simulink model "simulator_prototype"  (R2021b)
settings: Solver=VariableStepAuto  StartTime=0.0  StopTime=200  FixedStep=0.01  RelTol=1e-3
StopFcn:
  | run('simulate_robot_plot3.m')
(part 3 of 12)

== matlab function simulator_prototype/Kinematic Model/foward_kinematics ==
  data: q1 input; fk0_6 output; q2 input; q3 input; q4 input; q5 input; q6 input
function fk0_6 = foward_kinematics(q1,q2,q3,q4,q5,q6)
%#codegen

%    This function was generated by the Symbolic Math Toolbox version 9.0.
%    10-Oct-2021 02:08:10

t2 = cos(q1);
t3 = cos(q2);
t4 = cos(q4);
t5 = cos(q5);
t6 = cos(q6);
t7 = sin(q1);
t8 = sin(q2);
t9 = sin(q4);
t10 = sin(q5);
t11 = sin(q6);
t12 = q1+q2;
t23 = 9.007199254740992e+15;
t13 = cos(t12);
t14 = sin(t12);
t20 = t2.*1.051339e-1;
t21 = t7.*1.051339e-1;
t22 = t7.*3.235525e-2;
t24 = t2.*3.235525e-2;
t26 = t2.*t3.*3.641522e-2;
t27 = t2.*t8.*3.641522e-2;
t28 = t3.*t7.*3.641522e-2;
t29 = t7.*t8.*3.641522e-2;
t30 = t7.*t8.*2.462267e-2;
t32 = t2.*t3.*2.462267e-2;
t33 = t2.*t8.*2.462267e-2;
t34 = t3.*t7.*2.462267e-2;
t38 = (q3.*t23)./9.007199254740992e+15;
t41 = q3.*t23.*1.110223024625157e-16i;
t15 = t14.*7.742227997977903e+15;
t16 = t13.*4.602992943936994e+15;
t17 = t14.*4.602992943936994e+15;
t18 = t13.*7.742227997977903e+15;
t25 = -t22;
t31 = -t26;
t35 = -t30;
t39 = cos(t38);
t40 = sin(t38);
t42 = exp(t41);
t43 = -t41;
t19 = -t17;
t36 = t15+t16;
t44 = 1.0./t42;
t45 = t4.*t39;
t46 = t9.*t39;
t47 = t40.*1i;
t48 = t42-1.0;
t53 = t39.*7.38843356682345e-1;
t54 = t39.*2.61156643317655e-1;
t56 = t23.*t40.*9.543032792050485e-17;
t57 = t4.*t23.*t40.*5.673626844500105e-17;
t58 = t9.*t23.*t40.*5.673626844500105e-17;
t62 = t5.*t23.*t40.*(-9.543032792050485e-17);
t65 = t4.*t23.*t40.*(t17-t18).*(-1.232595164407831e-32);
t67 = t9.*t23.*t40.*(t17-t18).*(-1.232595164407831e-32);
t68 = (t4.*t23.*t40.*(t17-t18))./8.112963841460668e+31;
t69 = (t9.*t23.*t40.*(t17-t18))./8.112963841460668e+31;
t70 = t23.*t40.*5.540299264978165e-18;
t37 = t18+t19;
t49 = -t47;
t50 = t48.^2;
t52 = t39+t47-1.0;
t59 = t5.*t56;
t60 = t10.*t56;
t61 = -t58;
t63 = (t4.*t23.*t36.*t40)./8.112963841460668e+31;
t64 = (t9.*t23.*t36.*t40)./8.112963841460668e+31;
t71 = t53+2.61156643317655e-1;
t72 = t54+7.38843356682345e-1;
t77 = t46+t57;
t51 = t39+t49;
t55 = t52.^2;
t66 = -t64;
t73 = t13.*t71;
t74 = t13.*t72;
t75 = t14.*t71;
t76 = t14.*t72;
t78 = t45+t61;
t79 = t5.*t78;
t80 = t10.*t78;
t81 = t13.*t51.*t55.*2.196325630278387e-1;
t82 = t14.*t51.*t55.*2.196325630278387e-1;
t83 = -t81;
t84 = -t82;
t85 = t60+t79;
t86 = t62+t80;
t87 = t74+t82;
t88 = t75+t81;
t89 = t73+t84;
t90 = t76+t83;
t91 = t4.*t87;
t92 = t5.*t88;
t93 = t9.*t87;
t94 = t10.*t88;
t95 = t4.*t90;
t96 = t5.*t89;
t97 = t9.*t90;
t98 = t10.*t89;
t100 = t63+t93;
t101 = t66+t91;
t99 = -t95;
t102 = t67+t95;
t103 = t68+t97;
t104 = t5.*t100;
t105 = t10.*t100;
t106 = t69+t99;
t107 = -t104;
t108 = t5.*t103;
t109 = t10.*t103;
t111 = t92+t105;
t110 = -t109;
t112 = t94+t107;
t113 = t98+t108;
t114 = t96+t110;
et1 = t21+t24-t2.*t3.*5.561103841189621e-2;
et2 = t2.*t8.*3.603517512464e-2;
et3 = t3.*t7.*3.603517512464e-2;
et4 = t7.*t8.*5.561103841189621e-2;
et5 = t2.*t3.*t39.*6.463878411896211e-3;
et6 = t2.*t8.*t39.*1.087223487536e-2;
et7 = t3.*t7.*t39.*1.087223487536e-2;
et8 = t7.*t8.*t39.*(-6.463878411896211e-3);
et9 = t20+t25+t2.*t3.*3.603517512464e-2;
et10 = t2.*t8.*5.561103841189621e-2;
et11 = t3.*t7.*5.561103841189621e-2;
et12 = t7.*t8.*(-3.603517512464e-2);
et13 = t2.*t3.*t39.*1.087223487536e-2;
et14 = t2.*t8.*t39.*(-6.463878411896211e-3);
et15 = t3.*t7.*t39.*(-6.463878411896211e-3);
et16 = t7.*t8.*t39.*(-1.087223487536e-2);
et17 = t21+t24-t2.*t3.*7.464911842399381e-2;
et18 = t2.*t8.*4.735389991350965e-2;
et19 = t3.*t7.*4.735389991350965e-2;
et20 = t7.*t8.*7.464911842399381e-2;
et21 = t2.*t3.*t39.*2.550195842399381e-2;
et22 = t2.*t8.*t39.*4.289426008649035e-2;
et23 = t3.*t7.*t39.*4.289426008649035e-2;
et24 = t7.*t8.*t39.*(-2.550195842399381e-2);
et25 = t20+t25+t2.*t3.*4.735389991350965e-2;
et26 = t2.*t8.*7.464911842399381e-2;
et27 = t3.*t7.*7.464911842399381e-2;
et28 = t7.*t8.*(-4.735389991350965e-2);
et29 = t2.*t3.*t39.*4.289426008649035e-2;
et30 = t2.*t8.*t39.*(-2.550195842399381e-2);
et31 = t3.*t7.*t39.*(-2.550195842399381e-2);
et32 = t7.*t8.*t39.*(-4.289426008649035e-2);
et33 = t21+t24+t29+t31+t33+t34-t74.*1.273194e-2+t75.*6.562549e-2+t92.*(3.0./5.0e+2)+t105.*(3.0./5.0e+2)+t13.*t44.*t50.*1.44134945686578e-2;
et34 = t14.*t44.*t50.*(-2.79634861451666e-3);
et35 = t20+t25+t27+t28+t32+t35+t73.*6.562549e-2+t76.*1.273194e-2+t96.*(3.0./5.0e+2)-t109.*(3.0./5.0e+2)-t13.*t44.*t50.*2.79634861451666e-3;
et36 = t14.*t44.*t50.*(-1.44134945686578e-2);
mt1 = [t2,t13,t87,t101,t101,-t11.*t111-t6.*(t64-t91),0.0,0.0,t23.*t40.*5.673626844500105e-17,t77,t77,t6.*t77+t11.*t86,-t7,-t14,-t76+t81,t106,t106,-t6.*t102-t11.*t114,0.0,0.0,0.0,0.0,0.0,0.0,0.0,0.0,t23.*t36.*t40.*(-1.232595164407831e-32),-t100,t112,t112,1.0,1.0,t39,t78,t85,t85,0.0,0.0];
mt2 = [(t23.*t40.*(t17-t18))./8.112963841460668e+31,t103,t113,t113,0.0,0.0,0.0,0.0,0.0,0.0,t7,t14,t88,t88,t111,t6.*t111-t11.*(t64-t91),0.0,0.0,t56,t56,t59-t80,t11.*t77-t6.*t86,t2,t13,t89,t89,t114,-t11.*t102+t6.*t114,0.0,0.0,0.0,0.0,0.0,0.0,0.0,t21+t24,t21+t24+t29+t31+t33+t34,et1+et2+et3+et4+et5+et6+et7+et8,et17+et18+et19+et20+et21+et22+et23+et24,et33+et34,0.0,0.0,0.0];
mt3 = [t23.*t40.*1.404277280157545e-18,t70,t70-t80.*(3.0./5.0e+2)+t5.*t23.*t40.*5.725819675230291e-19,0.0,t20+t25,t20+t25+t27+t28+t32+t35,et9+et10+et11+et12+et13+et14+et15+et16,et25+et26+et27+et28+et29+et30+et31+et32,et35+et36,1.0,1.0,1.0,1.0,1.0,1.0];
fk0_6 = reshape([mt1,mt2,mt3],6,16);

== matlab function simulator_prototype/Kinematic Model/MATLAB Function ==
  data: fk_0_6 input; coord output
function coord = fcn(fk_0_6)
    coord = zeros(size(fk_0_6, 1),3);
    for i = 1:size(fk_0_6, 1)
        h_i = reshape(fk_0_6(i,:),4,4);
        coord(i,:) = real(h_i(1:3,4)');
    end

end

== matlab function simulator_prototype/Dynamic Model/Gravity_vector ==
  data: q1 input; tau_g output; q2 input; q3 input; q4 input; q5 input; q6 input
function tau_g = Gravity_vector(q1,q2,q3,q4,q5,q6)
%#codegen

%    This function was generated by the Symbolic Math Toolbox version 9.0.
%    08-Oct-2021 20:02:44

t2 = conj(q1);
t3 = conj(q2);
t4 = conj(q3);
t5 = conj(q4);
t6 = conj(q5);
t7 = conj(q6);
t23 = atan(5.945307920587191e-1);
t24 = 9.007199254740992e+15;
t8 = cos(t2);
t9 = cos(t3);
t10 = cos(t5);
t11 = cos(t6);
t12 = cos(t7);
t13 = sin(t2);
t14 = sin(t3);
t15 = sin(t5);
t16 = sin(t6);
t17 = sin(t7);
t18 = t2+t3;
t28 = (t4.*t24)./9.007199254740992e+15;
t31 = t4.*t24.*1.110223024625157e-16i;
t19 = cos(t18);
t20 = sin(t18);
t25 = t18+t23;
t29 = cos(t28);
t30 = sin(t28);
t32 = -t31;
t33 = exp(t31);
t21 = t19.*4.602992943936994e+15;
t22 = t20.*7.742227997977903e+15;
t26 = sin(t25);
t34 = -t29;
t35 = exp(t32);
t36 = t30.*1i;
t37 = t10.*t29;
t38 = t15.*t29;
t45 = t29.*7.38843356682345e-1;
t46 = t29.*2.61156643317655e-1;
t49 = t10.*t24.*t30.*5.673626844500105e-17;
t50 = t15.*t24.*t30.*5.673626844500105e-17;
t51 = t11.*t24.*t30.*9.543032792050485e-17;
t65 = t8.*t9.*t29.*4.598452461113469e-3;
t66 = t13.*t14.*t29.*4.598452461113469e-3;
t68 = t8.*t14.*t29.*7.73459091191916e-3;
t69 = t9.*t13.*t29.*7.73459091191916e-3;
t27 = t21+t22;
t39 = t35-1.0;
t41 = t15.*t26.*t30;
t42 = t10.*t26.*t30;
t44 = t29+t36;
t47 = t34+t36+1.0;
t52 = -t50;
t53 = -t51;
t61 = t45+2.61156643317655e-1;
t62 = t46+7.38843356682345e-1;
t67 = -t65;
t70 = -t68;
t71 = -t69;
t72 = t38+t49;
t40 = t39.^2;
t43 = -t41;
t48 = t47.^2;
t54 = t42.*1.834077274308e-6;
t56 = t41.*1.663769266031448e-3;
t57 = (t10.*t24.*t27.*t30)./8.112963841460668e+31;
t58 = (t15.*t24.*t27.*t30)./8.112963841460668e+31;
t63 = t19.*t62;
t64 = t20.*t61;
t73 = t37+t52;
t55 = -t54;
t59 = -t56;
t60 = -t58;
t74 = t16.*t73;
t75 = t20.*t33.*t40.*1.993592526573721e-4;
t76 = t63.*9.0769442339979e-4;
t77 = t64.*1.123016940370151e-2;
t78 = t19.*t33.*t40.*1.027576994682181e-3;
t81 = t20.*t44.*t48.*2.196325630278387e-1;
t82 = t19.*t44.*t48.*2.196325630278387e-1;
t84 = t19.*t44.*t48.*1.438933894689597e-3;
t79 = -t77;
t80 = -t78;
t83 = t53+t74;
t85 = -t84;
t86 = t63+t81;
t87 = t64+t82;
t88 = t10.*t86;
t89 = t11.*t87;
t90 = t15.*t86;
t91 = t16.*t87.*1.33075164870018e-3;
t92 = -t91;
t93 = t90.*1.834077274308e-6;
t95 = t88.*1.663769266031448e-3;
t96 = t89.*1.03455776890854e-3;
t98 = t42+t90;
t99 = t43+t88;
t102 = t12.*(t41-t88).*(-7.12549896598485e-4);
t103 = t57+t90;
t104 = t60+t88;
t105 = t17.*(t41-t88).*(-1.31098441441266e-3);
t106 = t17.*(t41-t88).*1.31098441441266e-3;
t94 = -t93;
t97 = -t96;
t100 = t16.*t98;
t101 = t11.*t98.*1.33075164870018e-3;
t108 = t16.*t103;
t107 = t100.*1.03455776890854e-3;
t110 = t89+t100;
t115 = t89+t108;
t109 = -t107;
t111 = t17.*t110.*7.12549896598485e-4;
t113 = t12.*t110.*1.31098441441266e-3;
t112 = -t111;
t114 = -t113;
et1 = t8.*(-1.504629097027635e-2)-t13.*3.4643831698033e-2;
et2 = t19.*4.486342129859745e-3-t20.*3.161090981652867e-3+t55+t59+t66+t67+t70+t71+t75+t76+t79+t80+t85+t92+t94+t95+t97+t101+t102+t106+t109+t112+t114;
et3 = t8.*t9.*2.789883597074818e-2;
et4 = t8.*t14.*(-1.805586507105727e-2);
et5 = t9.*t13.*(-1.805586507105727e-2);
et6 = t13.*t14.*(-2.789883597074818e-2);
et7 = t19.*(-1.035229938014282e-2)+t20.*7.294263179826428e-3+t55+t59+t66+t67+t70+t71+t75+t76+t79+t80+t85+t92+t94+t95+t97+t101+t102+t106+t109+t112+t114;
et8 = t8.*t9.*2.716427583908298e-2;
et9 = t8.*t14.*(-1.753829165813497e-2);
et10 = t9.*t13.*(-1.753829165813497e-2);
et11 = t13.*t14.*(-2.716427583908298e-2);
et12 = t37.*-6.451751339289925e+65-t38.*5.852657213932193e+68;
et13 = t11.*t37.*4.681197925536181e+68-t12.*t38.*2.506543652270432e+68;
et14 = t16.*t37.*-3.639273854285582e+68+t24.*t30.*6.584058839489303e+53;
et15 = t17.*t38.*4.611662534593243e+68-t10.*t24.*t30.*3.320579308062288e+52+t11.*t24.*t30.*3.472970973069927e+52;
et16 = t12.*t16.*t37.*-4.611662534593243e+68+t15.*t24.*t30.*3.660482959263482e+49;
et17 = t16.*t17.*t37.*-2.506543652270432e+68+t16.*t24.*t30.*4.467282530947048e+52-t10.*t12.*t24.*t30.*1.422119335243286e+52;
et18 = t11.*t12.*t24.*t30.*4.400924679349397e+52-t11.*t15.*t24.*t30.*2.655937021474028e+52+t10.*t17.*t24.*t30.*2.616485235404362e+52;
et19 = t11.*t17.*t24.*t30.*2.392002826832272e+52+t15.*t16.*t24.*t30.*2.064788183416204e+52+t12.*t15.*t16.*t24.*t30.*2.616485235404362e+52;
et20 = t15.*t16.*t17.*t24.*t30.*1.422119335243286e+52;
et21 = t8.*t9.*t10.*5.058701277356498e-7;
et22 = t8.*t9.*t15.*4.539519387384721e-4;
et23 = t8.*t10.*t14.*8.508728807534787e-7;
et24 = t9.*t10.*t13.*8.508728807534787e-7;
et25 = t8.*t14.*t15.*7.635465560438749e-4;
et26 = t9.*t13.*t15.*7.635465560438749e-4;
et27 = t10.*t13.*t14.*(-5.058701277356498e-7);
et28 = t13.*t14.*t15.*(-4.539519387384721e-4);
et29 = t8.*t9.*t10.*t11.*5.84552790715085e-4;
et30 = t8.*t9.*t10.*t16.*(-4.544451487714901e-4);
et31 = t8.*t10.*t11.*t14.*9.832170150362058e-4;
et32 = t9.*t10.*t11.*t13.*9.832170150362058e-4;
et33 = t8.*t9.*t12.*t15.*(-3.129983201502934e-4);
et34 = t8.*t10.*t14.*t16.*(-7.643761346621835e-4);
et35 = t9.*t10.*t13.*t16.*(-7.643761346621835e-4);
et36 = t10.*t11.*t13.*t14.*(-5.84552790715085e-4);
et37 = t8.*t9.*t15.*t17.*5.758697340540054e-4;
et38 = t8.*t12.*t14.*t15.*(-5.264627574064825e-4);
et39 = t9.*t12.*t13.*t15.*(-5.264627574064825e-4);
et40 = t10.*t13.*t14.*t16.*4.544451487714901e-4;
et41 = t8.*t14.*t15.*t17.*9.686121253028882e-4;
et42 = t9.*t13.*t15.*t17.*9.686121253028882e-4;
et43 = t12.*t13.*t14.*t15.*3.129983201502934e-4;
et44 = t13.*t14.*t15.*t17.*(-5.758697340540054e-4);
et45 = t8.*t9.*t10.*t33.*(-2.529350638678249e-7);
et46 = t8.*t9.*t10.*t35.*(-2.529350638678249e-7);
et47 = t8.*t9.*t15.*t33.*(-2.269759693692361e-4);
et48 = t8.*t10.*t14.*t33.*1.503776838607606e-7;
et49 = t9.*t10.*t13.*t33.*1.503776838607606e-7;
et50 = t8.*t9.*t15.*t35.*(-2.269759693692361e-4);
et51 = t8.*t10.*t14.*t35.*1.503776838607606e-7;
et52 = t9.*t10.*t13.*t35.*1.503776838607606e-7;
et53 = t8.*t14.*t15.*t33.*1.349442028473875e-4;
et54 = t9.*t13.*t15.*t33.*1.349442028473875e-4;
et55 = t10.*t13.*t14.*t33.*2.529350638678249e-7;
et56 = t8.*t14.*t15.*t35.*1.349442028473875e-4;
et57 = t9.*t13.*t15.*t35.*1.349442028473875e-4;
et58 = t10.*t13.*t14.*t35.*2.529350638678249e-7;
et59 = t13.*t14.*t15.*t33.*2.269759693692361e-4;
et60 = t13.*t14.*t15.*t35.*2.269759693692361e-4;
et61 = t8.*t9.*t10.*t12.*t16.*(-5.758697340540054e-4);
et62 = t8.*t9.*t10.*t16.*t17.*(-3.129983201502934e-4);
et63 = t8.*t10.*t12.*t14.*t16.*(-9.686121253028882e-4);
et64 = t9.*t10.*t12.*t13.*t16.*(-9.686121253028882e-4);
et65 = t8.*t10.*t14.*t16.*t17.*(-5.264627574064825e-4);
et66 = t9.*t10.*t13.*t16.*t17.*(-5.264627574064825e-4);
et67 = t10.*t12.*t13.*t14.*t16.*5.758697340540054e-4;
et68 = t10.*t13.*t14.*t16.*t17.*3.129983201502934e-4;
et69 = t8.*t9.*t10.*t11.*t33.*(-2.922763953575425e-4);
et70 = t8.*t9.*t10.*t11.*t35.*(-2.922763953575425e-4);
et71 = t8.*t9.*t10.*t16.*t33.*2.272225743857451e-4;
et72 = t8.*t10.*t11.*t14.*t33.*1.737673168319871e-4;
et73 = t9.*t10.*t11.*t13.*t33.*1.737673168319871e-4;
et74 = t8.*t9.*t12.*t15.*t33.*1.564991600751467e-4;
et75 = t8.*t9.*t10.*t16.*t35.*2.272225743857451e-4;
et76 = t8.*t10.*t11.*t14.*t35.*1.737673168319871e-4;
et77 = t9.*t10.*t11.*t13.*t35.*1.737673168319871e-4;
et78 = t8.*t9.*t12.*t15.*t35.*1.564991600751467e-4;
et79 = t8.*t10.*t14.*t16.*t33.*(-1.350908171231782e-4);
et80 = t9.*t10.*t13.*t16.*t33.*(-1.350908171231782e-4);
et81 = t10.*t11.*t13.*t14.*t33.*2.922763953575425e-4;
et82 = t8.*t9.*t15.*t17.*t33.*(-2.879348670270027e-4);
et83 = t8.*t12.*t14.*t15.*t33.*(-9.304356959600123e-5);
et84 = t9.*t12.*t13.*t15.*t33.*(-9.304356959600123e-5);
et85 = t8.*t10.*t14.*t16.*t35.*(-1.350908171231782e-4);
et86 = t9.*t10.*t13.*t16.*t35.*(-1.350908171231782e-4);
et87 = t10.*t11.*t13.*t14.*t35.*2.922763953575425e-4;
et88 = t8.*t9.*t10.*t24.*t33.*4.931051864161687e-20i;
et89 = t8.*t9.*t15.*t17.*t35.*(-2.879348670270027e-4);
et90 = t8.*t12.*t14.*t15.*t35.*(-9.304356959600123e-5);
et91 = t9.*t12.*t13.*t15.*t35.*(-9.304356959600123e-5);
et92 = t8.*t9.*t10.*t24.*t35.*-4.931051864161687e-20i;
et93 = t10.*t13.*t14.*t16.*t33.*(-2.272225743857451e-4);
et94 = t8.*t14.*t15.*t17.*t33.*1.711861445548859e-4;
et95 = t9.*t13.*t15.*t17.*t33.*1.711861445548859e-4;
et96 = t12.*t13.*t14.*t15.*t33.*(-1.564991600751467e-4);
et97 = t10.*t13.*t14.*t16.*t35.*(-2.272225743857451e-4);
et98 = t8.*t9.*t15.*t24.*t33.*-5.495013069724294e-23i;
et99 = t8.*t10.*t14.*t24.*t33.*-2.931662170482671e-20i;
et100 = t8.*t14.*t15.*t17.*t35.*1.711861445548859e-4;
et101 = t9.*t10.*t13.*t24.*t33.*-2.931662170482671e-20i;
et102 = t9.*t13.*t15.*t17.*t35.*1.711861445548859e-4;
et103 = t12.*t13.*t14.*t15.*t35.*(-1.564991600751467e-4);
et104 = t8.*t9.*t15.*t24.*t35.*5.495013069724294e-23i;
et105 = t8.*t10.*t14.*t24.*t35.*2.931662170482671e-20i;
et106 = t9.*t10.*t13.*t24.*t35.*2.931662170482671e-20i;
et107 = t13.*t14.*t15.*t17.*t33.*2.879348670270027e-4;
et108 = t8.*t14.*t15.*t24.*t33.*3.266954472716198e-23i;
et109 = t9.*t13.*t15.*t24.*t33.*3.266954472716198e-23i;
et110 = t10.*t13.*t14.*t24.*t33.*-4.931051864161687e-20i;
et111 = t13.*t14.*t15.*t17.*t35.*2.879348670270027e-4;
et112 = t8.*t14.*t15.*t24.*t35.*-3.266954472716198e-23i;
et113 = t9.*t13.*t15.*t24.*t35.*-3.266954472716198e-23i;
et114 = t10.*t13.*t14.*t24.*t35.*4.931051864161687e-20i;
et115 = t13.*t14.*t15.*t24.*t33.*5.495013069724294e-23i;
et116 = t13.*t14.*t15.*t24.*t35.*-5.495013069724294e-23i;
et117 = t8.*t9.*t10.*t12.*t16.*t33.*2.879348670270027e-4;
et118 = t8.*t9.*t10.*t12.*t16.*t35.*2.879348670270027e-4;
et119 = t8.*t9.*t10.*t16.*t17.*t33.*1.564991600751467e-4;
et120 = t8.*t10.*t12.*t14.*t16.*t33.*(-1.711861445548859e-4);
et121 = t9.*t10.*t12.*t13.*t16.*t33.*(-1.711861445548859e-4);
et122 = t8.*t9.*t10.*t16.*t17.*t35.*1.564991600751467e-4;
et123 = t8.*t10.*t12.*t14.*t16.*t35.*(-1.711861445548859e-4);
et124 = t9.*t10.*t12.*t13.*t16.*t35.*(-1.711861445548859e-4);
et125 = t8.*t9.*t10.*t12.*t24.*t33.*-3.399943514605762e-20i;
et126 = t8.*t9.*t10.*t12.*t24.*t35.*3.399943514605762e-20i;
et127 = t8.*t10.*t14.*t16.*t17.*t33.*(-9.304356959600123e-5);
et128 = t9.*t10.*t13.*t16.*t17.*t33.*(-9.304356959600123e-5);
et129 = t10.*t12.*t13.*t14.*t16.*t33.*(-2.879348670270027e-4);
et130 = t8.*t9.*t11.*t15.*t24.*t33.*-6.349703310810532e-20i;
et131 = t8.*t10.*t14.*t16.*t17.*t35.*(-9.304356959600123e-5);
et132 = t9.*t10.*t13.*t16.*t17.*t35.*(-9.304356959600123e-5);
et133 = t10.*t12.*t13.*t14.*t16.*t35.*(-2.879348670270027e-4);
et134 = t8.*t9.*t10.*t17.*t24.*t33.*6.255383628303558e-20i;
et135 = t8.*t10.*t12.*t14.*t24.*t33.*2.021371110693469e-20i;
et136 = t9.*t10.*t12.*t13.*t24.*t33.*2.021371110693469e-20i;
et137 = t8.*t9.*t11.*t15.*t24.*t35.*6.349703310810532e-20i;
et138 = t8.*t9.*t10.*t17.*t24.*t35.*-6.255383628303558e-20i;
et139 = t8.*t10.*t12.*t14.*t24.*t35.*-2.021371110693469e-20i;
et140 = t9.*t10.*t12.*t13.*t24.*t35.*-2.021371110693469e-20i;
et141 = t10.*t13.*t14.*t16.*t17.*t33.*(-1.564991600751467e-4);
et142 = t8.*t9.*t15.*t16.*t24.*t33.*4.936409356982393e-20i;
et143 = t8.*t11.*t14.*t15.*t24.*t33.*3.775094138714057e-20i;
et144 = t9.*t11.*t13.*t15.*t24.*t33.*3.775094138714057e-20i;
et145 = t10.*t13.*t14.*t16.*t17.*t35.*(-1.564991600751467e-4);
et146 = t8.*t10.*t14.*t17.*t24.*t33.*-3.719018183166459e-20i;
et147 = t9.*t10.*t13.*t17.*t24.*t33.*-3.719018183166459e-20i;
et148 = t10.*t12.*t13.*t14.*t24.*t33.*3.399943514605762e-20i;
et149 = t8.*t9.*t15.*t16.*t24.*t35.*-4.936409356982393e-20i;
et150 = t8.*t11.*t14.*t15.*t24.*t35.*-3.775094138714057e-20i;
et151 = t9.*t11.*t13.*t15.*t24.*t35.*-3.775094138714057e-20i;
et152 = t8.*t10.*t14.*t17.*t24.*t35.*3.719018183166459e-20i;
et153 = t9.*t10.*t13.*t17.*t24.*t35.*3.719018183166459e-20i;
et154 = t10.*t12.*t13.*t14.*t24.*t35.*-3.399943514605762e-20i;
et155 = t8.*t14.*t15.*t16.*t24.*t33.*-2.934847364932814e-20i;
et156 = t9.*t13.*t15.*t16.*t24.*t33.*-2.934847364932814e-20i;
et157 = t11.*t13.*t14.*t15.*t24.*t33.*6.349703310810532e-20i;
et158 = t10.*t13.*t14.*t17.*t24.*t33.*-6.255383628303558e-20i;
et159 = t8.*t14.*t15.*t16.*t24.*t35.*2.934847364932814e-20i;
et160 = t9.*t13.*t15.*t16.*t24.*t35.*2.934847364932814e-20i;
et161 = t11.*t13.*t14.*t15.*t24.*t35.*-6.349703310810532e-20i;
et162 = t10.*t13.*t14.*t17.*t24.*t35.*6.255383628303558e-20i;
et163 = t13.*t14.*t15.*t16.*t24.*t33.*-4.936409356982393e-20i;
et164 = t13.*t14.*t15.*t16.*t24.*t35.*4.936409356982393e-20i;
et165 = t8.*t9.*t12.*t15.*t16.*t24.*t33.*6.255383628303558e-20i;
et166 = t8.*t9.*t12.*t15.*t16.*t24.*t35.*-6.255383628303558e-20i;
et167 = t8.*t9.*t15.*t16.*t17.*t24.*t33.*3.399943514605762e-20i;
et168 = t8.*t12.*t14.*t15.*t16.*t24.*t33.*-3.719018183166459e-20i;
et169 = t9.*t12.*t13.*t15.*t16.*t24.*t33.*-3.719018183166459e-20i;
et170 = t8.*t9.*t15.*t16.*t17.*t24.*t35.*-3.399943514605762e-20i;
et171 = t8.*t12.*t14.*t15.*t16.*t24.*t35.*3.719018183166459e-20i;
et172 = t9.*t12.*t13.*t15.*t16.*t24.*t35.*3.719018183166459e-20i;
et173 = t8.*t14.*t15.*t16.*t17.*t24.*t33.*-2.021371110693469e-20i;
et174 = t9.*t13.*t15.*t16.*t17.*t24.*t33.*-2.021371110693469e-20i;
et175 = t12.*t13.*t14.*t15.*t16.*t24.*t33.*-6.255383628303558e-20i;
et176 = t8.*t14.*t15.*t16.*t17.*t24.*t35.*2.021371110693469e-20i;
et177 = t9.*t13.*t15.*t16.*t17.*t24.*t35.*2.021371110693469e-20i;
et178 = t12.*t13.*t14.*t15.*t16.*t24.*t35.*6.255383628303558e-20i;
et179 = t13.*t14.*t15.*t16.*t17.*t24.*t33.*-3.399943514605762e-20i;
et180 = t13.*t14.*t15.*t16.*t17.*t24.*t35.*3.399943514605762e-20i;
et181 = t63.*1.273194e-2-t64.*6.562549e-2-t88.*6.48e-5-t89.*3.131399999999998e-4-t108.*3.131399999999998e-4;
et182 = t8.*t9.*(-3.823389842399381e-2);
et183 = t8.*t14.*2.273122991350965e-2;
et184 = t9.*t13.*2.273122991350965e-2;
et185 = t13.*t14.*3.823389842399381e-2+t16.*t87.*1.247162e-2-t11.*t103.*1.247162e-2;
et186 = t12.*t115.*(-1.838876e-2)-t17.*t115.*9.99471e-3-t12.*(t58-t88).*9.99471e-3+t17.*(t58-t88).*1.838876e-2;
et187 = t8.*t9.*t29.*2.550195842399381e-2;
et188 = t8.*t14.*t29.*4.289426008649035e-2;
et189 = t9.*t13.*t29.*4.289426008649035e-2;
et190 = t13.*t14.*t29.*(-2.550195842399381e-2);
et191 = t19.*t33.*t40.*(-1.44134945686578e-2);
et192 = t20.*t33.*t40.*2.79634861451666e-3+t15.*t24.*t27.*t30.*7.987216665362745e-37;
et193 = t38.*6.48e-5-t74.*3.131399999999998e-4-t11.*t73.*1.247162e-2-t12.*t72.*9.99471e-3+t17.*t72.*1.838876e-2;
et194 = t12.*(t51-t74).*1.838876e-2+t17.*(t51-t74).*9.99471e-3+t10.*t24.*t30.*3.676510195236068e-21;
et195 = t11.*t24.*t30.*2.988305288502687e-20-t16.*t24.*t30.*1.190170786299927e-18;
mt1 = [et1+et2+et3+et4+et5+et6,et7+et8+et9+et10+et11,t24.*cos(t25).*(et12+et13+et14+et15+et16+et17+et18+et19+et20).*(-3.156096247042585e-88)];
mt2 = [et21+et22+et23+et24+et25+et26+et27+et28+et29+et30+et31+et32+et33+et34+et35+et36+et37+et38+et39+et40+et41+et42+et43+et44+et45+et46+et47+et48+et49+et50+et51+et52+et53+et54+et55+et56+et57+et58+et59+et60+et61+et62+et63+et64+et65+et66+et67+et68+et69+et70+et71+et72+et73+et74+et75+et76+et77+et78+et79+et80+et81+et82+et83+et84+et85+et86+et87+et88+et89+et90+et91+et92+et93+et94+et95+et96+et97+et98+et99+et100+et101+et102+et103+et104+et105+et106+et107+et108+et109+et110+et111+et112+et113+et114+et115+et116+et117+et118+et119+et120+et121+et122+et123+et124+et125+et126+et127+et128+et129+et130+et131+et132+et133+et134+et135+et136+et137+et138+et139+et140+et141+et142+et143+et144+et145+et146+et147+et148+et149+et150+et151+et152+et153+et154+et155+et156+et157+et158+et159+et160+et161+et162+et163+et164+et165+et166+et167+et168+et169+et170+et171+et172+et173+et174+et175+et176+et177+et178+et179+et180];
mt3 = [t72.*(et181+et182+et183+et184+et185+et186+et187+et188+et189+et190+et191+et192).*7.12927035e-2-(t58-t88).*(et193+et194+et195).*7.12927035e-2,0.0];
tau_g = real(reshape([mt1,mt2,mt3],6,1));

== matlab function simulator_prototype/Dynamic Model/Dissipative_vector ==
  data: dq1 input; tau_d output; dq2 input; dq3 input; dq4 input; dq5 input; dq6 input
function tau_d = Dissipative_vector(dq1,dq2, dq3, dq4, dq5, dq6)
%#codegen

%    This function was generated by the Symbolic Math Toolbox version 9.0.
%    08-Oct-2021 20:02:47
tau_d = real([conj(dq1)./1.0e+1;conj(dq2)./1.0e+1;conj(dq3)./1.0e+1;conj(dq4)./1.0e+1;conj(dq5)./1.0e+1;conj(dq6)./1.0e+1]);
